simulink model "Target_Control_System"  (R2021b)
settings: Solver=FixedStepDiscrete  StartTime=0.0  StopTime=5  RelTol=1e-3
PreLoadFcn:
  | RTWConfigurationCB('preloadfcn', bdroot);
PostLoadFcn:
  | load('configuration/data_struct.mat');
  | load('configuration/fluxMaps_propMotor.mat');
  | load('configuration/parameterInit_PROP.mat');
  | load('configuration/parameterInit_PUMP.mat');
  | load('configuration/parameterInit_PITCH.mat');
  | load('configuration/parameterInit_TILT.mat');
  | %load('configuration/base_workspace_signal_definition.mat');
  | %load('resolvedatastores_to_baseworkspace_for_faster_simulation.mat');
model workspace (MAT data in the model file):
  SIMULATION_OPTIONS : Simulink.Parameter (value not decoded)
  TARGET_CODE_GEN : Simulink.Parameter (value not decoded)
  TCS_SAMPLE_FREQ_HZ : Simulink.Parameter (value not decoded)
symbols that are objects in the model workspace (value not decoded): TARGET_CODE_GEN, TCS_SAMPLE_FREQ_HZ
undefined symbols (not defined in the file): A_DQ_REF_LPF_INIT__PITCH, A_DQ_REF_LPF_INIT__PROP, A_DQ_REF_LPF_INIT__PUMP, A_DQ_REF_LPF_INIT__TILT, A_OBSERVER_CONFIDENCE_INIT__PITCH, A_OBSERVER_CONFIDENCE_INIT__PROP, A_OBSERVER_CONFIDENCE_INIT__PUMP, A_OBSERVER_CONFIDENCE_INIT__TILT, ACTUATOR_MAX_ANGLE_TRIP__PITCH, ACTUATOR_MIN_ANGLE_TRIP__PITCH, ACTUATOR_POS_SENSOR_INV_DIRECTION__PITCH, ACTUATOR_POS_SENSOR_INV_DIRECTION__TILT, ACTUATOR_POS_SENSOR_OFFSET__PITCH, ACTUATOR_POS_SENSOR_OFFSET__TILT, ADC_scaler1_baseaddr_TILT, ADC_SCALER_FLOAT_TO_FIXPOINT_EXPANSION, ANGLE_ELEC_FROM_SENSOR_OFFSET_INIT__PITCH, ANGLE_ELEC_FROM_SENSOR_OFFSET_INIT__PROP, ANGLE_ELEC_FROM_SENSOR_OFFSET_INIT__PUMP, ANGLE_ELEC_FROM_SENSOR_OFFSET_INIT__TILT, AUTO_CLEAR_FAULTS_ENABLED__PITCH, AUTO_CLEAR_FAULTS_ENABLED__PROP, AUTO_CLEAR_FAULTS_ENABLED__PUMP, AUTO_CLEAR_FAULTS_ENABLED__TILT, AUTO_CLEAR_FAULTS_WAIT_TICKS__PITCH, AUTO_CLEAR_FAULTS_WAIT_TICKS__PROP, AUTO_CLEAR_FAULTS_WAIT_TICKS__PUMP, AUTO_CLEAR_FAULTS_WAIT_TICKS__TILT, AUTO_I_ZERO_IDLE_TICKS__PITCH, AUTO_I_ZERO_IDLE_TICKS__PROP, AUTO_I_ZERO_IDLE_TICKS__PUMP, AUTO_I_ZERO_IDLE_TICKS__TILT, AUTO_I_ZERO_OFFSET_IDC_THRESHOLD__PITCH, AUTO_I_ZERO_OFFSET_IDC_THRESHOLD__PROP, AUTO_I_ZERO_OFFSET_IDC_THRESHOLD__PUMP, AUTO_I_ZERO_OFFSET_IDC_THRESHOLD__TILT, AUTO_I_ZERO_OFFSET_IPH_THRESHOLD__PITCH, AUTO_I_ZERO_OFFSET_IPH_THRESHOLD__PROP, AUTO_I_ZERO_OFFSET_IPH_THRESHOLD__PUMP, AUTO_I_ZERO_OFFSET_IPH_THRESHOLD__TILT, AUTO_SENSORLESS_SWITCHOVER_DISABLE_OMEGA, AUTO_SENSORLESS_SWITCHOVER_ENABLE_OMEGA, AUTO_SENSORLESS_SWITCHOVER_MIN_CONFIDENCE, AUXILIARY_PROTECTION_UNIT_BASEADDR__TILT, blanking_max_error_omega_INIT_PITCH, blanking_max_error_omega_INIT_TILT, blanking_max_error_position_INIT_PITCH, blanking_max_error_position_INIT_TILT, BRUTE_START_I_Q_REF_RAMP_SPEED__PITCH, BRUTE_START_I_Q_REF_RAMP_SPEED__PROP, BRUTE_START_I_Q_REF_RAMP_SPEED__PUMP, BRUTE_START_I_Q_REF_RAMP_SPEED__TILT, CONTROL_LOOP_DT_INIT__PITCH, CONTROL_LOOP_DT_INIT__PROP, CONTROL_LOOP_DT_INIT__PUMP, CONTROL_LOOP_DT_INIT__TILT, CORRECTION_FILTER_SCALE__PITCH, CORRECTION_FILTER_SCALE__PROP, CORRECTION_FILTER_SCALE__PUMP, CORRECTION_FILTER_SCALE__TILT ... (+458)
libraries: simulink x178, Reusables_Lib x24
(part 43 of 47)

== stateflow chart Target_Control_System/MainLoop/pumpMotor_mainLoop/motorStateMachineLogic(&oPump)/Idle-Loop State Machine Pump ==
  state InitialState
  state State_90
    //startup delay
    state Wait_Ticks_
    state Startup_Delay_
      entry:
      oPump.oMot_.oState_.uiDriveState_ = 95;
      oPump.oMot_.oOut_.uiLastFaultState_ = 0;
    (default) -> State_90.Wait_Ticks_
    State_90.Wait_Ticks_ -> Startup_Delay_ : [after(35, tick)]
  state State_246
    // Second phase of voltage nulling
    state Wait_uiDelayTicks_
    state Next
      entry:
      oPump.oMot_.oState_.uiDriveState_ = 100;
      oPump.oMot_.oOut_.uiEnableGateDrive_ = 0x0;
      oPump.oMot_.oIn_.uiVoltageOffsetNullingActive_ = 0;
    (default) -> State_246.Wait_uiDelayTicks_
    State_246.Wait_uiDelayTicks_ -> State_246.Next : [after(25, tick)]
  state State_95
    // Current offset nulling
    state Wait_Ticks_
    state Current_offset_nulling
      entry:
      oPump.oMot_.oState_.uiCurrentOffsetNullingPerformed_++;
      oPump.oMot_.oIn_.uiCurrentOffsetNullingActive_ = 0;
      oPump.oMot_.oIn_.uiVoltageOffsetNullingActive_ = 0;
      oPump.oMot_.oState_.uiDriveState_ = 99;
      //SZ: still need to re-write the FPGA protection to enable the sum of current detection for fault 1034
    (default) -> State_95.Wait_Ticks_
    State_95.Wait_Ticks_ -> Current_offset_nulling : [after(6, tick)]
  state State_245
    // Initial phase of voltage nulling
    state Wait_uiDelayTicks_
    state Next
      entry:
      oPump.oMot_.oState_.uiDriveState_ = 246;
    (default) -> State_245.Wait_uiDelayTicks_
    State_245.Wait_uiDelayTicks_ -> State_245.Next : [after(25, tick)]
  state State_99
    // Minimum command set not met. Also the return state after clearing trips etc.
    state Substate
    state Idle_state
      entry:
      oPump.oMot_.oState_.uiDriveState_ = 100;
    state Cleanup
      // We somehow left the forced angle start sequence without cleaning up.
      // Clean up now.
      entry:
      oPump.oMot_.oState_.oRampDataOmegaERef_.oParam_.fUpslope_ = oPump.oMot_.oState_.fForcedAngleStartOrigOmegaRamp_;
      oPump.oMot_.oState_.oRampDataOmegaERef_.fSetpoint_ = fabs(oPump.oMot_.oState_.fForcedAngleStartOrigOmega_);
      oPump.oMot_.oState_.uiSpeedControllerActive_ = oPump.oMot_.oState_.uiForcedAngleStartOrigSpeedControllerActive_;
      oPump.oMot_.oState_.oRampDataIqRef_.oParam_.fUpslope_ = oPump.oMot_.oState_.fForcedAngleStartOrigIRamp_;
      oPump.oMot_.oState_.oRampDataIqRef_.oParam_.fDownslope_ = oPump.oMot_.oState_.oRampDataIqRef_.oParam_.fUpslope_;
      oPump.oMot_.oOut_.uiForcedAngle_ = 0;
      oPump.oMot_.oState_.uiForcedAngleStartParametersSet_ = 0;
    (default) -> State_99.Substate
    State_99.Substate -> (junction 251)
    (junction 251) -> Idle_state [order 2] : [!oPump.oMot_.oState_.uiMinimumCommandSetFlags_]
    (junction 251) -> State_99.Cleanup [order 1] : [oPump.oMot_.oState_.uiForcedAngleStartParametersSet_]
    State_99.Cleanup -> Idle_state : [!oPump.oMot_.oState_.uiMinimumCommandSetFlags_]
  state State_104
    // Idle, motor spinning (windmilling, coasting down),
    // autostart enabled, and a nonzero current applied
    // Removed autostart functionality
    entry:
    oPump.oMot_.oState_.uiDriveState_ = 102;
  state State_224
    state Transition_220
      // Direction or confidence check failed, restart full sequence
      entry:
      oPump.oMot_.oState_.uiDriveState_ = 220;
    state FlyingStart
      entry:
      oPump.oMot_.oOut_.uiPwmDutyTicksFromMainA_ = uint32((oPump.oMot_.oParam_.fPwmPeriodTicksMainloopFloat_)/2);
      oPump.oMot_.oOut_.uiPwmDutyTicksFromMainB_ = uint32((oPump.oMot_.oParam_.fPwmPeriodTicksMainloopFloat_)/2);
      oPump.oMot_.oOut_.uiPwmDutyTicksFromMainC_ = uint32((oPump.oMot_.oParam_.fPwmPeriodTicksMainloopFloat_)/2);
      oPump.oMot_.oState_.oRampDataOmegaERef_.fRampOut_ = oPump.oMot_.oIn_.fOmegaEObserverLpf2_;
      oPump.oMot_.oState_.oRampDataIqRef_.fRampOut_ = 0.0;
      oPump.oIsr_.oParam_.oPiDataIq_.fState_ = 0.0F;
      oPump.oIsr_.oParam_.oPiDataId_.fState_ = 0.0F;
      oPump.oMot_.oParam_.oPiDataRpm_.fState_ = 0.0F;
      oPump.oMot_.oParam_.oPid2DataRpmCtrl_.fState_ = 0.0F;
      oPump.oMot_.oState_.uiDriveState_ = 200;
      // release gate signals
      oPump.oMot_.oOut_.uiEnableGateDrive_ = 0x7;
      // Release control in main interrupt
      oPump.oMot_.oOut_.uiCurrentControllerActive_ = 1;
    state uiAutomaticFanControlMode_
      entry:
      oPump.oMot_.oState_.uiDriveState_ = 205;
    (default) -> (junction 274)
    (junction 274) -> (junction 275) [order 2]
    (junction 274) -> (junction 276) [order 1] : [oPump.oMot_.oState_.fObserverConfidence_ > oPump.oMot_.oParam_.fSlaveStartMinConfidence_ && ....
        | !(oPump.oMot_.oOut_.fOmegaEObserverXlpf2_ * oPump.oMot_.oState_.fForcedAngleStartDirection_ < 0.0F)]
        | // The faster we go, the further we jump in the sequence
        | // [SZ]: need to investigate implementing the __signbitf() function in Stateflow]
    (junction 275) -> State_224.Transition_220
    (junction 276) -> FlyingStart : //Confidence wise we're good to go, but is the speed high enough?
        | [fabs(oPump.oMot_.oOut_.fOmegaEObserverXlpf2_) > ....
        |  (oPump.oMot_.oParam_.fSlaveStartMinOmegaE_)]
    FlyingStart -> State_224.uiAutomaticFanControlMode_ : [oPump.oMot_.oParam_.uiAutomaticFanControlMode_ == 1]
  state State_103
    // Idle, motor not spinning, autostart enabled, and a nonzero current applied
    // Removed autostart functionality
    entry:
    oPump.oMot_.oState_.uiDriveState_ = 101;
  state State_100
    //Idle, determine if the motor is externally driven (e.g. windmilling or spindown) or standing still
    state Initialization
      entry:
      oPump.oMot_.oState_.oRampDataOmegaERef_.fRampOut_ = 0.0;
      oPump.oMot_.oState_.oRampDataIqRef_.fRampOut_ = 0.0;
    state Entering_State_101
      entry:
      oPump.oMot_.oState_.uiDriveState_ = 101;
    state Cleanup
      // We somehow left the forced angle start sequence without cleaning up.
      // Clean up now.
      entry:
      oPump.oMot_.oState_.uiDriveState_  = 99;
    state Entering_State_102
      entry:
      oPump.oMot_.oState_.uiDriveState_ = 102;
    state pwm50PercentDuty
      //Pre-set 50% duty
      entry:
      oPump.oMot_.oOut_.uiPwmRequestFromMain_ = 1;
      oPump.oMot_.oOut_.uiPwmDutyTicksFromMainA_ = cast(((oPump.oMot_.oParam_.fPwmPeriodTicksMainloopFloat_) / 2), uint32);
      oPump.oMot_.oOut_.uiPwmDutyTicksFromMainB_ = cast(((oPump.oMot_.oParam_.fPwmPeriodTicksMainloopFloat_) / 2), uint32);
      oPump.oMot_.oOut_.uiPwmDutyTicksFromMainC_ = cast(((oPump.oMot_.oParam_.fPwmPeriodTicksMainloopFloat_) / 2), uint32);
    (default) -> State_100.Initialization
    State_100.Initialization -> (junction 189)
    (junction 189) -> (junction 186) [order 2]
    (junction 186) -> Entering_State_101 [order 1] : [(fabs(oPump.oMot_.oOut_.fOmegaEObserverXlpf2_) < oPump.oMot_.oParam_.fFlyingStartOmegaELimit_) ....
        |  || (oPump.oMot_.oState_.fObserverConfidence_ < 0.7F)]
    (junction 189) -> State_100.Cleanup [order 1] : [oPump.oMot_.oState_.uiMinimumCommandSetFlags_]
    (junction 186) -> Entering_State_102 [order 2]
    Entering_State_101 -> pwm50PercentDuty
    Entering_State_102 -> pwm50PercentDuty
  state State_102
    // Idle, motor spinning by external means (windmilling, downhill, large inertia, ....)
    state Stay_at_102
      entry:
      oPump.oMot_.oState_.uiDriveState_ = 102;
    state Transition_to_101
      entry:
      oPump.oMot_.oState_.uiDriveState_ = 101;
    (default) -> (junction 192)
    (junction 192) -> Stay_at_102 [order 2]
    (junction 192) -> Transition_to_101 [order 1] : [fabs(oPump.oMot_.oOut_.fOmegaEObserverXlpf2_) < oPump.oMot_.oParam_.fFlyingStartOmegaELimit_ ....
        | || oPump.oMot_.oState_.fObserverConfidence_ < 0.65F]
  state State_222
    state Transition_224
      entry:
      oPump.oMot_.oState_.uiDriveState_ = 224;
    state Transition_223
      entry:
      oPump.oMot_.oState_.uiDriveState_ = 223;
    state Transition_220
      // Direction or confidence check failed, restart full sequence
      entry:
      oPump.oMot_.oState_.uiDriveState_ = 220;
    (default) -> (junction 301)
    (junction 301) -> (junction 302) [order 2]
    (junction 301) -> (junction 304) [order 1] : [oPump.oMot_.oState_.fObserverConfidence_ > oPump.oMot_.oParam_.fSlaveStartMinConfidence_ && ....
        | !(oPump.oMot_.oOut_.fOmegaEObserverXlpf2_ * oPump.oMot_.oState_.fForcedAngleStartDirection_ < 0.0F)]
        | // The faster we go, the further we jump in the sequence
        | // [SZ]: need to investigate implementing the __signbitf() function in Stateflow]
    (junction 302) -> State_222.Transition_220
    (junction 304) -> (junction 303) [order 1]
    (junction 303) -> State_222.Transition_224 : [fabs(oPump.oMot_.oOut_.fOmegaEObserverXlpf2_) >....
        |  (oPump.oMot_.oParam_.fSlaveStartMinOmegaE_)]
    (junction 304) -> State_222.Transition_223 [order 2]
  state State_223
    state Transition_220
      // Direction or confidence check failed, restart full sequence
      entry:
      oPump.oMot_.oState_.uiDriveState_ = 220;
    state Transition_224
      entry:
      oPump.oMot_.oState_.uiDriveState_ = 224;
    (default) -> (junction 263)
    (junction 263) -> (junction 264) [order 2]
    (junction 263) -> (junction 265) [order 1] : [oPump.oMot_.oState_.fObserverConfidence_ > oPump.oMot_.oParam_.fSlaveStartMinConfidence_ && ....
        | !(oPump.oMot_.oOut_.fOmegaEObserverXlpf2_ * oPump.oMot_.oState_.fForcedAngleStartDirection_ < 0.0F)]
        | // The faster we go, the further we jump in the sequence
        | // [SZ]: need to investigate implementing the __signbitf() function in Stateflow]
    (junction 264) -> State_223.Transition_220
    (junction 265) -> State_223.Transition_224 : [fabs(oPump.oMot_.oOut_.fOmegaEObserverXlpf2_) >....
        |  (oPump.oMot_.oParam_.fSlaveStartMinOmegaE_)]
  state State_101
    // Idle, motor not spinning
    state Initialization
      entry:
      oPump.oMot_.oState_.oRampDataOmegaERef_.fRampOut_ = 0.0;
      oPump.oMot_.oState_.oRampDataIqRef_.fRampOut_ = 0.0;
    state Transition_to_102
      entry:
      oPump.oMot_.oState_.uiDriveState_ = 102;
    (default) -> State_101.Initialization
    State_101.Initialization -> (junction 227)
    (junction 227) -> Transition_to_102 [order 1] : [(fabs(oPump.oMot_.oOut_.fOmegaEObserverXlpf2_) > oPump.oMot_.oParam_.fFlyingStartOmegaELimit_) ....
        | && (oPump.oMot_.oState_.fObserverConfidence_ > 0.65F)]
  state State_220
    // Flying start, first of multiple stages.
    // There has to be an uninterrupted chain of OKs. Too low confidence at any step,
    // and fall back to this initial state.
    state Substate
    state Transition_224
      entry:
      oPump.oMot_.oState_.uiDriveState_ = 224;
    state Transition_223
      entry:
      oPump.oMot_.oState_.uiDriveState_ = 223;
    state Transition_222
      entry:
      oPump.oMot_.oState_.uiDriveState_ = 222;
    state Transition_221
      /* Don't check for the speed for the slowest
      //advancement path, that will happen in state 224 */
      entry:
      oPump.oMot_.oState_.uiDriveState_ = 221;
    (default) -> State_220.Substate
    State_220.Substate -> (junction 346)
    (junction 346) -> (junction 348) : [oPump.oMot_.oState_.fObserverConfidence_ > oPump.oMot_.oParam_.fSlaveStartMinConfidence_ && ....
        | !(oPump.oMot_.oOut_.fOmegaEObserverXlpf2_ * oPump.oMot_.oState_.fForcedAngleStartDirection_ < 0.0F)]
        | // The faster we go, the further we jump in the sequence
        | // [SZ]: need to investigate implementing the __signbitf() function in Stateflow]
    (junction 348) -> (junction 347) [order 1]
    (junction 348) -> (junction 349) [order 3]
    (junction 349) -> (junction 350) [order 2]
    (junction 347) -> State_220.Transition_224 : [fabs(oPump.oMot_.oOut_.fOmegaEObserverXlpf2_) >....
        |  (oPump.oMot_.oParam_.fSlaveStartMinOmegaE_)]
    (junction 348) -> State_220.Transition_223 [order 2] : [fabs(4.0F * oPump.oMot_.oOut_.fOmegaEObserverXlpf2_) >....
        |  (3.0F * oPump.oMot_.oParam_.fSlaveStartMinOmegaE_)]
    (junction 349) -> State_220.Transition_222 [order 1] : [fabs(2.0F * oPump.oMot_.oOut_.fOmegaEObserverXlpf2_) >....
        |  (oPump.oMot_.oParam_.fSlaveStartMinOmegaE_)]
    (junction 350) -> Transition_221
  state State_221
    state Transition_224
      entry:
      oPump.oMot_.oState_.uiDriveState_ = 224;
    state Transition_223
      entry:
      oPump.oMot_.oState_.uiDriveState_ = 223;
    state Transition_222
      entry:
      oPump.oMot_.oState_.uiDriveState_ = 222;
    state Transition_220
      // Direction or confidence check failed, restart full sequence
      entry:
      oPump.oMot_.oState_.uiDriveState_ = 220;
    (default) -> (junction 298)
    (junction 298) -> (junction 328) [order 2]
    (junction 298) -> (junction 330) [order 1] : [oPump.oMot_.oState_.fObserverConfidence_ > oPump.oMot_.oParam_.fSlaveStartMinConfidence_ && ....
        | !(oPump.oMot_.oOut_.fOmegaEObserverXlpf2_ * oPump.oMot_.oState_.fForcedAngleStartDirection_ < 0.0F)]
        | // The faster we go, the further we jump in the sequence
        | // [SZ]: need to investigate implementing the __signbitf() function in Stateflow]
    (junction 328) -> State_221.Transition_220
    (junction 330) -> (junction 329) [order 1]
    (junction 330) -> (junction 331) [order 3]
    (junction 329) -> State_221.Transition_224 : [fabs(oPump.oMot_.oOut_.fOmegaEObserverXlpf2_) >....
        |  (oPump.oMot_.oParam_.fSlaveStartMinOmegaE_)]
    (junction 330) -> State_221.Transition_223 [order 2] : [fabs(4.0F * oPump.oMot_.oOut_.fOmegaEObserverXlpf2_) >....
        |  (3.0F * oPump.oMot_.oParam_.fSlaveStartMinOmegaE_)]
    (junction 331) -> State_221.Transition_222
  state State_212
    // Forced angle. Current and speed are ramping.
    // Once we reach a certain predefined speed, turn off forced angle
    // (idea: look at observer confidence instead, or additionally)
    state Wait_RPM
      exit:
      // To avoid a sudden step in angle, add an offset to the estimated angle to give the forced angle. It'll ramp to zero
      //oPump.oMot_.oState_.oRampDataFluxMstrAngFrcd2clsdSmoothn_.fRampOut_ = oPump.oIsr_.oState_.fFluxMasterAngle_ - oPump.oIsr_.oState_.fFluxMainAngleRaw2_;
    state Restore_values
      // Restore values: (Mind the order of setting things, in case the interrupt starts halfway through)
      state Reset
        entry:
        oPump.oMot_.oOut_.uiForcedAngle_ = 0;
        oPump.oMot_.oState_.oRampDataOmegaERef_.oParam_.fUpslope_ = oPump.oMot_.oState_.fForcedAngleStartOrigOmegaRamp_;
        // The downslope wasn't touched in the first place, as forced angle start only relies on the upslope
        oPump.oMot_.oState_.uiDriveState_ = 213;
      (default) -> (junction 434)
      (junction 434) -> (junction 437) [order 1] : [oPump.oMot_.oState_.oRampDataFluxMstrAngFrcd2clsdSmoothn_.fRampOut_> PI_F]
          | {oPump.oMot_.oState_.oRampDataFluxMstrAngFrcd2clsdSmoothn_.fRampOut_ -= TWO_PI_F;}
      (junction 437) -> Reset [order 2]
      (junction 434) -> Reset [order 3]
      (junction 434) -> Reset [order 2] : [oPump.oMot_.oState_.oRampDataFluxMstrAngFrcd2clsdSmoothn_.fRampOut_ < -PI_F]
          | {oPump.oMot_.oState_.oRampDataFluxMstrAngFrcd2clsdSmoothn_.fRampOut_ += TWO_PI_F;}
      (junction 437) -> Reset [order 1] : [oPump.oMot_.oState_.oRampDataFluxMstrAngFrcd2clsdSmoothn_.fRampOut_ < -PI_F]
          | {oPump.oMot_.oState_.oRampDataFluxMstrAngFrcd2clsdSmoothn_.fRampOut_ += TWO_PI_F;}
    (default) -> Wait_RPM
    Wait_RPM -> Restore_values : [oPump.oMot_.oState_.oRampDataOmegaERef_.fRampOut_ > oPump.oMot_.oParam_.fForcedAngleOmegaEHandoff_ ]
  state State_213
    // Almost the end of forced angle
    state Wait_uiForcedStartPostTicks_
      exit:
      oPump.oMot_.oState_.oRampDataIqRef_.oParam_.fUpslope_ = oPump.oMot_.oState_.fForcedAngleStartOrigIRamp_;	// TODO whatabout downslope
      oPump.oMot_.oState_.oRampDataIqRef_.oParam_.fDownslope_ = oPump.oMot_.oState_.oRampDataIqRef_.oParam_.fUpslope_;
      oPump.oMot_.oState_.uiForcedAngleStartParametersSet_ = 0;
      oPump.oMot_.oState_.uiDriveState_ = 200;
    state uiAutomaticFanControlMode_
      entry:
      oPump.oMot_.oState_.uiDriveState_ = 205;
    (default) -> Wait_uiForcedStartPostTicks_
    Wait_uiForcedStartPostTicks_ -> (junction 409) : [after(oPump.oMot_.oParam_.uiForcedStartPostTicks_, tick)]
    (junction 409) -> (junction 406) [order 2]
    (junction 409) -> State_213.uiAutomaticFanControlMode_ [order 1] : [oPump.oMot_.oParam_.uiAutomaticFanControlMode_ == 1]
    State_213.uiAutomaticFanControlMode_ -> (junction 406)
  state State_211
    // Forced angle start, ramping the current while holding speed at zero.
    // After some time, we release the speed
    state Wait_uiForcedAngleSpeedDelayTicks_
    state Speed_loop_active
      entry:
      oPump.oMot_.oState_.oRampDataOmegaERef_.fSetpoint_ = oPump.oMot_.oState_.fForcedAngleStartOrigOmega_;
    state Speed_loop_inactive
      // Torque control. We don't actually know if the current is enough to reach the handoff point
      // So, we set the speedref to a bit above the handoff point. Past the handoff, this value becomes irrelevant.
      entry:
      oPump.oMot_.oState_.oRampDataOmegaERef_.fSetpoint_ = oPump.oMot_.oParam_.fForcedAngleOmegaEHandoff_ * 1.1F;
    state Bidirection
      // allow for clock and counterclockwise dir depending on current setpoint
      entry:
      oPump.oMot_.oState_.oRampDataOmegaERef_.fSetpoint_ = abs(oPump.oMot_.oState_.oRampDataOmegaERef_.fSetpoint_) * oPump.oMot_.oState_.fForcedAngleStartDirection_;
      oPump.oMot_.oState_.uiDriveState_ = 212;
    (default) -> Wait_uiForcedAngleSpeedDelayTicks_
    Wait_uiForcedAngleSpeedDelayTicks_ -> (junction 375) : [after(oPump.oMot_.oParam_.uiForcedAngleSpeedDelayTicks_, tick)]
    (junction 375) -> Speed_loop_active [order 1] : [oPump.oMot_.oState_.uiSpeedControllerActive_ == 1]
    (junction 375) -> Speed_loop_inactive [order 2]
    Speed_loop_active -> Bidirection
    Speed_loop_inactive -> Bidirection
  (default) -> InitialState
  InitialState -> State_90 [order 1] : [oPump.oMot_.oState_.uiDriveState_ == 90]
  State_90 -> InitialState : [!(oPump.oMot_.oState_.uiDriveState_ == 90)]
  InitialState -> State_246 [order 12] : [oPump.oMot_.oState_.uiDriveState_ == 246]
  State_246 -> InitialState : [!(oPump.oMot_.oState_.uiDriveState_ == 246)]
  InitialState -> State_95 [order 2] : [oPump.oMot_.oState_.uiDriveState_ == 95]
  Current_offset_nulling -> InitialState : [!(oPump.oMot_.oState_.uiDriveState_ == 95)]
  InitialState -> State_245 [order 11] : [oPump.oMot_.oState_.uiDriveState_ == 245]
  State_245 -> InitialState : [!(oPump.oMot_.oState_.uiDriveState_ == 245)]
  InitialState -> State_99 [order 3] : [oPump.oMot_.oState_.uiDriveState_ == 99]
  State_99 -> InitialState : [!(oPump.oMot_.oState_.uiDriveState_ == 99)]
  InitialState -> State_104 [order 8] : [oPump.oMot_.oState_.uiDriveState_ == 104]
  State_104 -> InitialState
  InitialState -> State_103 [order 7] : [oPump.oMot_.oState_.uiDriveState_ == 103]
  State_103 -> InitialState
  InitialState -> State_102 [order 6] : [oPump.oMot_.oState_.uiDriveState_ == 102]
  Stay_at_102 -> InitialState
  State_100.Cleanup -> InitialState
  Transition_to_101 -> InitialState
  pwm50PercentDuty -> InitialState
  InitialState -> State_100 [order 4] : [oPump.oMot_.oState_.uiDriveState_ == 100]
  InitialState -> State_101 [order 5] : [oPump.oMot_.oState_.uiDriveState_ == 101]
  State_224 -> (junction 293) : [!(oPump.oMot_.oState_.uiDriveState_ == 224)]
  (junction 293) -> State_224 [order 4] : [oPump.oMot_.oState_.uiDriveState_ == 224]
  State_223 -> (junction 293) : [!(oPump.oMot_.oState_.uiDriveState_ == 223)]
  (junction 293) -> State_223 [order 3] : [oPump.oMot_.oState_.uiDriveState_ == 223]
  State_222 -> (junction 293) : [!(oPump.oMot_.oState_.uiDriveState_ == 222)]
  (junction 322) -> State_222 [order 2] : [oPump.oMot_.oState_.uiDriveState_ == 222]
  (junction 227) -> InitialState [order 2] : // We're staying at rest.
  Transition_to_102 -> InitialState
  InitialState -> (junction 293) [order 10] : [(oPump.oMot_.oState_.uiDriveState_ >= 220) && (oPump.oMot_.oState_.uiDriveState_ <= 224)]
  (junction 293) -> InitialState [order 5]
  (junction 293) -> (junction 322) [order 2]
  State_221 -> (junction 293) : [!(oPump.oMot_.oState_.uiDriveState_ == 221)]
  State_220 -> (junction 293) : [!(oPump.oMot_.oState_.uiDriveState_ == 220)]
  (junction 293) -> State_220 [order 1] : [oPump.oMot_.oState_.uiDriveState_ == 220]
  (junction 322) -> State_221 [order 1] : [oPump.oMot_.oState_.uiDriveState_ == 221]
  InitialState -> (junction 380) [order 9] : [oPump.oMot_.oState_.uiDriveState_ == 211]
  (junction 380) -> InitialState [order 4]
  (junction 406) -> (junction 380) : {oPump.oMot_.oState_.oRampDataIqRef_.oParam_.fUpslope_ = oPump.oMot_.oState_.fForcedAngleStartOrigIRamp_;
      |  oPump.oMot_.oState_.oRampDataIqRef_.oParam_.fDownslope_ = oPump.oMot_.oState_.oRampDataIqRef_.oParam_.fUpslope_;
      |  oPump.oMot_.oState_.uiForcedAngleStartParametersSet_ = 0;}
  State_212 -> (junction 380) : [!(oPump.oMot_.oState_.uiDriveState_ == 212)]
      | {oPump.oMot_.oState_.oRampDataOmegaERef_.oParam_.fUpslope_ = oPump.oMot_.oState_.fForcedAngleStartOrigOmegaRamp_;
      | oPump.oMot_.oState_.oRampDataOmegaERef_.fSetpoint_ = fabs(oPump.oMot_.oState_.fForcedAngleStartOrigOmega_);
      | oPump.oMot_.oState_.oRampDataOmegaERef_.fRampOut_ = oPump.oMot_.oOut_.fOmegaEObserverXlpf2_;  // For the speed controller, if used
      | oPump.oMot_.oState_.uiSpeedControllerActive_ = oPump.oMot_.oState_.uiForcedAngleStartOrigSpeedControllerActive_;
      | oPump.oMot_.oOut_.uiForcedAngle_ = 0;}
  (junction 380) -> State_212 [order 2] : [oPump.oMot_.oState_.uiDriveState_ == 212]
  (junction 380) -> State_213 [order 3] : [oPump.oMot_.oState_.uiDriveState_ == 213]
  State_211 -> (junction 380) : [!(oPump.oMot_.oState_.uiDriveState_ == 211)]
  (junction 380) -> State_211 [order 1] : [oPump.oMot_.oState_.uiDriveState_ == 211]
  data: oPump data_store_memory; PI_F constant single =3.14159265359; TWO_PI_F constant single =6.28318530718

== stateflow chart Target_Control_System/MainLoop/pumpMotor_mainLoop/Decimation gate A for 200 Hz Pump/Current offset nulling/initiateOffsetNulling(&oPump)/Chart ==
  state Start
  state initiateOffsetNulling
    //We can only do this if idle
    entry:
    oPump.oIsr_.oState_.fOffsetIntegratorIa_ = 0.0;
    oPump.oIsr_.oState_.fOffsetIntegratorIb_ = 0.0;
    oPump.oIsr_.oState_.fOffsetIntegratorIc_ = 0.0;
    oPump.oIsr_.oState_.fOffsetIntegratorIdc_ = 0.0;
    oPump.oMot_.oState_.uiDriveState_ = 95;
  (default) -> Start
  initiateOffsetNulling -> Start : [oPump.oMot_.oState_.uiCurrentOffsetNullingPerformed_ == 1]
  Start -> initiateOffsetNulling : [oPump.oMot_.oState_.uiDriveState_ >= 99 && ...
      | oPump.oMot_.oState_.uiDriveState_ < 102]
  data: oPump data_store_memory

== stateflow chart Target_Control_System/MainLoop/pitchMotor_mainLoop/Decimation gate for 10 Hz Pitch/Idle-Loop State Machine Pitch ==
  state InitialState
  state State_90
    //startup delay
    state Wait_Ticks_
    state Startup_Delay_
      entry:
      oPitch.oMot_.oState_.uiDriveState_ = 95;
      oPitch.oMot_.oOut_.uiLastFaultState_ = 0;
    (default) -> State_90.Wait_Ticks_
    State_90.Wait_Ticks_ -> Startup_Delay_ : [after(35, tick)]
  state State_246
    // Second phase of voltage nulling
    state Wait_uiDelayTicks_
    state Next
      entry:
      oPitch.oMot_.oState_.uiDriveState_ = 100;
      oPitch.oMot_.oOut_.uiEnableGateDrive_ = 0x0;
      oPitch.oMot_.oIn_.uiVoltageOffsetNullingActive_ = 0;
    (default) -> State_246.Wait_uiDelayTicks_
    State_246.Wait_uiDelayTicks_ -> State_246.Next : [after(25, tick)]
  state State_95
    // Current offset nulling
    state Wait_Ticks_
    state Current_offset_nulling
      entry:
      oPitch.oMot_.oState_.uiCurrentOffsetNullingPerformed_++;
      oPitch.oMot_.oIn_.uiCurrentOffsetNullingActive_ = 0;
      oPitch.oMot_.oIn_.uiVoltageOffsetNullingActive_ = 0;
      oPitch.oMot_.oState_.uiDriveState_ = 99;
      //SZ: still need to re-write the FPGA protection to enable the sum of current detection for fault 1034
    (default) -> State_95.Wait_Ticks_
    State_95.Wait_Ticks_ -> Current_offset_nulling : [after(6, tick)]
  state State_245
    // Initial phase of voltage nulling
    state Wait_uiDelayTicks_
    state Next
      entry:
      oPitch.oMot_.oState_.uiDriveState_ = 246;
    (default) -> State_245.Wait_uiDelayTicks_
    State_245.Wait_uiDelayTicks_ -> State_245.Next : [after(25, tick)]
  state State_99
    // Minimum command set not met. Also the return state after clearing trips etc.
    state Substate
    state Idle_state
      entry:
      oPitch.oMot_.oState_.uiDriveState_ = 100;
    state Cleanup
      // We somehow left the forced angle start sequence without cleaning up.
      // Clean up now.
      entry:
      oPitch.oMot_.oState_.oRampDataOmegaERef_.oParam_.fUpslope_ = oPitch.oMot_.oState_.fForcedAngleStartOrigOmegaRamp_;
      oPitch.oMot_.oState_.oRampDataOmegaERef_.fSetpoint_ = fabs(oPitch.oMot_.oState_.fForcedAngleStartOrigOmega_);
      oPitch.oMot_.oState_.uiSpeedControllerActive_ = oPitch.oMot_.oState_.uiForcedAngleStartOrigSpeedControllerActive_;
      oPitch.oMot_.oState_.oRampDataIqRef_.oParam_.fUpslope_ = oPitch.oMot_.oState_.fForcedAngleStartOrigIRamp_;
      oPitch.oMot_.oState_.oRampDataIqRef_.oParam_.fDownslope_ = oPitch.oMot_.oState_.oRampDataIqRef_.oParam_.fUpslope_;
      oPitch.oMot_.oOut_.uiForcedAngle_ = 0;
      oPitch.oMot_.oState_.uiForcedAngleStartParametersSet_ = 0;
    (default) -> Substate
    Substate -> (junction 251)
    (junction 251) -> Idle_state [order 2] : [!oPitch.oMot_.oState_.uiMinimumCommandSetFlags_]
    (junction 251) -> State_99.Cleanup [order 1] : [oPitch.oMot_.oState_.uiForcedAngleStartParametersSet_]
    State_99.Cleanup -> Idle_state : [!oPitch.oMot_.oState_.uiMinimumCommandSetFlags_]
  state State_104
    // Idle, motor spinning (windmilling, coasting down),
    // autostart enabled, and a nonzero current applied
    // Removed autostart functionality
    entry:
    oPitch.oMot_.oState_.uiDriveState_ = 102;
  state State_103
    // Idle, motor not spinning, autostart enabled, and a nonzero current applied
    // Removed autostart functionality
    entry:
    oPitch.oMot_.oState_.uiDriveState_ = 101;
  state State_100
    //Idle, determine if the motor is externally driven (e.g. windmilling or spindown) or standing still
    state Initialization
      entry:
      oPitch.oMot_.oState_.oRampDataOmegaERef_.fRampOut_ = 0.0;
      oPitch.oMot_.oState_.oRampDataIqRef_.fRampOut_ = 0.0;
    state Entering_State_101
      entry:
      oPitch.oMot_.oState_.uiDriveState_ = 101;
    state Cleanup
      // We somehow left the forced angle start sequence without cleaning up.
      // Clean up now.
      entry:
      oPitch.oMot_.oState_.uiDriveState_  = 99;
    state Entering_State_102
      entry:
      oPitch.oMot_.oState_.uiDriveState_ = 102;
    state pwm50PercentDuty
      //Pre-set 50% duty
      entry:
      oPitch.oMot_.oOut_.uiPwmRequestFromMain_ = 1;
      oPitch.oMot_.oOut_.uiPwmDutyTicksFromMainA_ = cast(((oPitch.oMot_.oParam_.fPwmPeriodTicksMainloopFloat_) / 2), uint32);
      oPitch.oMot_.oOut_.uiPwmDutyTicksFromMainB_ = cast(((oPitch.oMot_.oParam_.fPwmPeriodTicksMainloopFloat_) / 2), uint32);
      oPitch.oMot_.oOut_.uiPwmDutyTicksFromMainC_ = cast(((oPitch.oMot_.oParam_.fPwmPeriodTicksMainloopFloat_) / 2), uint32);
    (default) -> State_100.Initialization
    State_100.Initialization -> (junction 189)
    (junction 189) -> (junction 186) [order 2]
    (junction 186) -> Entering_State_101 [order 1] : [(fabs(oPitch.oMot_.oOut_.fOmegaEObserverXlpf2_) < oPitch.oMot_.oParam_.fFlyingStartOmegaELimit_) ....
        |  || (oPitch.oMot_.oState_.fObserverConfidence_ < 0.7F)]
    (junction 189) -> State_100.Cleanup [order 1] : [oPitch.oMot_.oState_.uiMinimumCommandSetFlags_]
    (junction 186) -> Entering_State_102 [order 2]
    Entering_State_101 -> pwm50PercentDuty
    Entering_State_102 -> pwm50PercentDuty
  state State_102
    // Idle, motor spinning by external means (windmilling, downhill, large inertia, ....)
    state Stay_at_102
      entry:
      oPitch.oMot_.oState_.uiDriveState_ = 102;
    state Transition_to_101
      entry:
      oPitch.oMot_.oState_.uiDriveState_ = 101;
    (default) -> (junction 192)
    (junction 192) -> Stay_at_102 [order 2]
    (junction 192) -> Transition_to_101 [order 1] : [fabs(oPitch.oMot_.oOut_.fOmegaEObserverXlpf2_) < oPitch.oMot_.oParam_.fFlyingStartOmegaELimit_ ....
        | || oPitch.oMot_.oState_.fObserverConfidence_ < 0.65F]
  state State_101
    // Idle, motor not spinning
    state Initialization
      entry:
      oPitch.oMot_.oState_.oRampDataOmegaERef_.fRampOut_ = 0.0;
      oPitch.oMot_.oState_.oRampDataIqRef_.fRampOut_ = 0.0;
    state Transition_to_102
      entry:
      oPitch.oMot_.oState_.uiDriveState_ = 102;
    (default) -> State_101.Initialization
    State_101.Initialization -> (junction 227)
    (junction 227) -> Transition_to_102 [order 1] : [(fabs(oPitch.oMot_.oOut_.fOmegaEObserverXlpf2_) > oPitch.oMot_.oParam_.fFlyingStartOmegaELimit_) ....
        | && (oPitch.oMot_.oState_.fObserverConfidence_ > 0.65F)]
  (default) -> InitialState
  InitialState -> State_90 [order 1] : [oPitch.oMot_.oState_.uiDriveState_ == 90]
  State_90 -> InitialState : [!(oPitch.oMot_.oState_.uiDriveState_ == 90)]
  InitialState -> State_246 [order 10] : [oPitch.oMot_.oState_.uiDriveState_ == 246]
  State_246 -> InitialState : [!(oPitch.oMot_.oState_.uiDriveState_ == 246)]
  InitialState -> State_95 [order 2] : [oPitch.oMot_.oState_.uiDriveState_ == 95]
  Current_offset_nulling -> InitialState : [!(oPitch.oMot_.oState_.uiDriveState_ == 95)]
  InitialState -> State_245 [order 9] : [oPitch.oMot_.oState_.uiDriveState_ == 245]
  State_245 -> InitialState : [!(oPitch.oMot_.oState_.uiDriveState_ == 245)]
  InitialState -> State_99 [order 3] : [oPitch.oMot_.oState_.uiDriveState_ == 99]
  State_99 -> InitialState : [!(oPitch.oMot_.oState_.uiDriveState_ == 99)]
  InitialState -> State_104 [order 8] : [oPitch.oMot_.oState_.uiDriveState_ == 104]
  State_104 -> InitialState
  InitialState -> State_103 [order 7] : [oPitch.oMot_.oState_.uiDriveState_ == 103]
  State_103 -> InitialState
  InitialState -> State_102 [order 6] : [oPitch.oMot_.oState_.uiDriveState_ == 102]
  Stay_at_102 -> InitialState
  State_100.Cleanup -> InitialState
  Transition_to_101 -> InitialState
  pwm50PercentDuty -> InitialState
  InitialState -> State_100 [order 4] : [oPitch.oMot_.oState_.uiDriveState_ == 100]
  InitialState -> State_101 [order 5] : [oPitch.oMot_.oState_.uiDriveState_ == 101]
  (junction 227) -> InitialState [order 2] : // We're staying at rest.
  Transition_to_102 -> InitialState
  data: oPitch data_store_memory; PI_F constant single =3.14159265359; TWO_PI_F constant single =6.28318530718

== stateflow chart Target_Control_System/MainLoop/pitchMotor_mainLoop/Decimation gate for 10 Hz Pitch/Function-Call Subsystem/DC_overvoltage_pitch ==
  state Start
  state Drive_trip
    // Disable the drive and enter a trip state (error state)
    entry:
    oPitch.oMot_.oOut_.uiEnableGateDrive_ = 0;
    oPitch.oMot_.oOut_.uiCurrentControllerActive_ = 0;
    // NOTE: the actual turning off is done in the ctrl interrupt
    // formerly: Xil_Out32(uiGateDriverBaseaddr_, 0x0);
  state Store_previous_fault
    // If we were already in a fault state, store the previous fault:
    entry:
    oPitch.oMot_.oOut_.uiLastFaultState_ = oPitch.oMot_.oState_.uiDriveState_;
  state setTripState
    entry:
    oPitch.oMot_.oState_.uiDriveState_ = Udc_tripCode;
  (default) -> Start
  Start -> (junction 26) [order 2] : [(oPitch.oMot_.oOut_.fUdcLpf_ > oPitch.oMot_.oParam_.fUdcMaxTrip_) && ...
      | oPitch.oMot_.oState_.uiDriveState_ > 0]
      | {Udc_tripCode = 1004;}
  Start -> (junction 26) [order 1] : [oPitch.oMot_.oOut_.fUdcLpf_ < oPitch.oMot_.oParam_.fUdcMinTrip_ && ...
      | (oPitch.oMot_.oState_.uiDriveState_ > 199 && oPitch.oMot_.oState_.uiDriveState_ < 1000)]
      | {Udc_tripCode = 1003;}
  setTripState -> Start
  (junction 26) -> Drive_trip [order 1] : [oPitch.oMot_.oState_.uiDriveState_ >= 200]
  (junction 26) -> (junction 31) [order 2]
  Drive_trip -> (junction 31)
  (junction 31) -> Store_previous_fault [order 1] : [oPitch.oMot_.oState_.uiDriveState_ >= 1000]
  (junction 31) -> setTripState [order 2]
  Store_previous_fault -> setTripState
  data: Udc_tripCode local single; oPitch data_store_memory

== stateflow chart Target_Control_System/MainLoop/tiltMotor_mainLoop/mainTask_tilt/motorTaskMainFastStep(&oTilt)/enableDrive(&oTilt) ==
  state Disabled
    state Default
    state Disable_Drive
      entry:
      oTilt.oMot_.oState_.uiDriveState_ = 100;
      oTilt.oMot_.oOut_.uiEnableGateDrive_ = 0x0;
      oTilt.oMot_.oOut_.uiCurrentControllerActive_ = 0;
    state Simulation
      entry:
      oTilt.oMot_.oState_.uiDriveState_ = 101;
      oTilt.oMot_.oOut_.uiEnableGateDrive_ = 0x0;
    (default) -> (junction 283)
    (junction 283) -> Default [order 3]
    (junction 283) -> Disable_Drive [order 2] : [oTilt.oMot_.oState_.uiDriveState_ >= 200 && ....
        |  oTilt.oMot_.oState_.uiDriveState_ <= 299]
    (junction 283) -> Simulation [order 1] : [TARGET_CODE_GEN ==0]
  state Position_hold_mode
    // Mostly intended for the VP. In position hold mode, the inverter will inject 0 RPM current in the motor to passively hold a motor in place.
    // The position sensors are not needed for this.
    // When issuing the enable command, the drive enters state 226, which is just for flagging, the inverters do not actually turn on.
    // (Use a special command for that.)
    entry:
    oTilt.oMot_.oState_.uiDriveState_ = 226;
    oTilt.oIsr_.oParam_.oPiDataIq_.fState_ = 0;
    oTilt.oIsr_.oParam_.oPiDataId_.fState_ = 0;
    // Pre-set 50% duty
    oTilt.oMot_.oOut_.uiPwmRequestFromMain_ = 1;
    oTilt.oMot_.oOut_.uiPwmDutyTicksFromMainA_ = uint32((oTilt.oMot_.oParam_.fPwmPeriodTicksMainloopFloat_)/2);
    oTilt.oMot_.oOut_.uiPwmDutyTicksFromMainB_ = uint32((oTilt.oMot_.oParam_.fPwmPeriodTicksMainloopFloat_)/2);
    oTilt.oMot_.oOut_.uiPwmDutyTicksFromMainC_ = uint32((oTilt.oMot_.oParam_.fPwmPeriodTicksMainloopFloat_)/2);
  state DC_undervoltage_trip
    state Fault_A
      entry:
      oTilt.oMot_.oOut_.uiCurrentControllerActive_ = 0;
      oTilt.oMot_.oOut_.uiEnableGateDrive_ = 0;
    state Fault_B
      // If we were already in a fault state, store the previous fault:
      entry:
      oTilt.oMot_.oOut_.uiLastFaultState_ = oTilt.oMot_.oState_.uiDriveState_;
    state Fault_C
      entry:
      oTilt.oMot_.oState_.uiDriveState_ = 1003;
    (default) -> (junction 164)
    (junction 164) -> Fault_A [order 1] : [oTilt.oMot_.oState_.uiDriveState_>= 200]
    (junction 164) -> (junction 271) [order 2]
    (junction 271) -> Fault_C [order 2]
    (junction 271) -> Fault_B [order 1] : [oTilt.oMot_.oState_.uiDriveState_>= 1000]
    Fault_B -> Fault_C
  state Slave_start
    // Slave start is not applicable to position control.
    // Not a position control inverter; slave role is set: Perform a slave start (wait for the motor to 'somehow' reach a minimum speed, then jump on).
    entry:
    // We have to set one item aside; the desired rotation direction, as signalled by the sign of the current
    oTilt.oMot_.oState_.fForcedAngleStartDirection_ = single(oTilt.oMot_.oIn_.fIqSetpoint_ >= 0);
    // in other areas of MBD, we use oPitch.oMot_.oState_.oRampDataIqRef_.fRampOut_...should we here?
    // Don't actually turn on the output stage, but instead, monitor the motor feedback.
    // Once confident, perform a running start.
    // The rest is handled via state machine.
    oTilt.oMot_.oState_.uiDriveState_ = 220;
  state Enabled
    // [SZ]: Still need to model the setupForFlyingStart() function, which involves calling NEON sin/cos functions in Stateflow
    state Open_loop_start
      // Open loop start from standstill. Risky, and rough on hardware
      state Open_loop_start_A
        entry:
        oTilt.oMot_.oState_.oRampDataFluxFeedforwardGain_.fRampOut_ = 0.0;
        oTilt.oMot_.oState_.oRampDataOmegaERef_.fRampOut_ = 0.0;
        oTilt.oMot_.oState_.oRampDataIqRef_.fRampOut_ = 0.0;
        oTilt.oMot_.oState_.uiDriveState_ = 200;
      state Open_loop_start_B
        entry:
        oTilt.oMot_.oState_.uiDriveState_ = 205;
      (default) -> Open_loop_start_A
      Open_loop_start_A -> Open_loop_start_B [order 1] : [oTilt.oMot_.oParam_.uiAutomaticFanControlMode_ == 1]
    state Standing_start
      // ----- Set up for forced angle start ----
      state Store_reference
        // Store original references and ramp rates aside:
        entry:
        oTilt.oMot_.oState_.fForcedAngleStartOrigIRamp_ = oTilt.oMot_.oState_.oRampDataIqRef_.oParam_.fUpslope_;
        // TODO: whatabout downslope?
        oTilt.oMot_.oState_.fForcedAngleStartOrigOmega_ = oTilt.oMot_.oState_.oRampDataOmegaERef_.fSetpoint_;
        oTilt.oMot_.oState_.fForcedAngleStartOrigOmegaRamp_ = oTilt.oMot_.oState_.oRampDataOmegaERef_.oParam_.fUpslope_;
        // The downslope is never touched, as it doesn't matter for forced angle start
        oTilt.oMot_.oState_.uiForcedAngleStartOrigSpeedControllerActive_ = oTilt.oMot_.oState_.uiSpeedControllerActive_;
        // We have to set one item aside; the desired rotation direction, as signalled by the sign of the current
        oTilt.oMot_.oState_.fForcedAngleStartDirection_ = single(oTilt.oMot_.oState_.oRampDataIqRef_.fRampOut_ >= 0);
        // should this be oPitch.oMot_.oIn_.fIqSetpoint_ >= 0; ??
      state Global_signal
        // Signals to the rest of the program.
        oTilt.oMot_.oOut_.uiForcedAngle_ = 1;
        oTilt.oMot_.oState_.uiDriveState_ = 211;
      state Initialization
        // Set up initial values
        entry:
        // Delete this section once the uiForcedAngleStartParametersSet_ flag is working properly...
        oTilt.oMot_.oState_.fForcedAngleStartOrigIRamp_ = oTilt.oMot_.oState_.oRampDataIqRef_.oParam_.fUpslope_;
        // TODO: whatabout downslope?
        oTilt.oMot_.oState_.fForcedAngleStartOrigOmega_ = oTilt.oMot_.oState_.oRampDataOmegaERef_.fSetpoint_;
        oTilt.oMot_.oState_.fForcedAngleStartOrigOmegaRamp_ = oTilt.oMot_.oState_.oRampDataOmegaERef_.oParam_.fUpslope_;
        // The downslope is never touched, as it doesn't matter for forced angle start
        oTilt.oMot_.oState_.uiForcedAngleStartOrigSpeedControllerActive_ = oTilt.oMot_.oState_.uiSpeedControllerActive_;
        // We have to set one item aside; the desired rotation direction, as signalled by the sign of the current
        oTilt.oMot_.oState_.fForcedAngleStartDirection_ = single(oTilt.oMot_.oState_.oRampDataIqRef_.fRampOut_ >= 0);
        oTilt.oMot_.oState_.fIqRefBeforeRamp_ = oTilt.oMot_.oParam_.fForcedAngleIRef_;
        //oTilt.oMot_.oState_.oRampDataIqRef_.oParam_.fUpslope_ = oTilt.oMot_.oParam_.fForcedAngleIRamp_;
        oTilt.oMot_.oState_.oRampDataIqRef_.oParam_.fUpslope_ = oTilt.oMot_.oParam_.fForcedAngleIRamp_*10*(TARGET_CODE_GEN==0)+...
        oTilt.oMot_.oParam_.fForcedAngleIRamp_*(TARGET_CODE_GEN==1); // Adjust for 100 Hz state machine in simulation
        oTilt.oMot_.oState_.oRampDataIqRef_.oParam_.fDownslope_ = oTilt.oMot_.oState_.oRampDataIqRef_.oParam_.fUpslope_;
        //oTilt.oMot_.oState_.oRampDataOmegaERef_.oParam_.fUpslope_ = oTilt.oMot_.oParam_.fForcedAngleOmegaERamp_;
        oTilt.oMot_.oState_.oRampDataOmegaERef_.oParam_.fUpslope_ = oTilt.oMot_.oParam_.fForcedAngleOmegaERamp_*10*(TARGET_CODE_GEN==0)+...
        oTilt.oMot_.oParam_.fForcedAngleOmegaERamp_*(TARGET_CODE_GEN==1); // Adjust for 100 Hz state machine in simulation
        oTilt.oMot_.oState_.oRampDataOmegaERef_.fRampOut_ = 0.0F;
        oTilt.oMot_.oState_.oRampDataOmegaERef_.fSetpoint_ = 0.0F;
        oTilt.oMot_.oState_.oRampDataIqRef_.fRampOut_ = 0.0F;
        oTilt.oMot_.oState_.uiSpeedControllerActive_ = 0;
        oTilt.oMot_.oState_.uiForcedAngleStartParametersSet_ = 1;
        oTilt.oMot_.oState_.oRampDataFluxFeedforwardGain_.fRampOut_ = 0.0F;
      (default) -> Global_signal
      Global_signal -> (junction 233)
      (junction 233) -> Store_reference [order 1] : [!(oTilt.oMot_.oState_.uiForcedAngleStartParametersSet_ == 1)]
      (junction 233) -> Initialization [order 2]
      Store_reference -> Initialization
    state Half_duty_preset
      // Pre-set 50% duty
      entry:
      oTilt.oMot_.oOut_.uiPwmRequestFromMain_ = 1;
      oTilt.oMot_.oOut_.uiPwmDutyTicksFromMainA_ = uint32((oTilt.oMot_.oParam_.fPwmPeriodTicksMainloopFloat_)/2);
      oTilt.oMot_.oOut_.uiPwmDutyTicksFromMainB_ = uint32((oTilt.oMot_.oParam_.fPwmPeriodTicksMainloopFloat_)/2);
      oTilt.oMot_.oOut_.uiPwmDutyTicksFromMainC_ = uint32((oTilt.oMot_.oParam_.fPwmPeriodTicksMainloopFloat_)/2);
      oTilt.oIsr_.oParam_.oPiDataIq_.fState_ = 0.0F;
      oTilt.oIsr_.oParam_.oPiDataId_.fState_ = 0.0F;
      oTilt.oMot_.oParam_.oPiDataRpm_.fState_ = 0.0F;
      oTilt.oMot_.oParam_.oPid2DataRpmCtrl_.fState_ = 0.0F;
      oTilt.oMot_.oState_.oPosSensor_.oPidDataPosCtrl_.fState_ = 0.0F;
      oTilt.oMot_.oState_.oRampDataPos_.fRampOut_ = oTilt.oMot_.oState_.oPosSensor_.oGbx_.fCurrentOutputAngle_;
      // Prevent jerk motions on start up.
      // [SZ]: Moved here to avoid the "Unconditional Path Out of State with During Actions or Child States" warning
    state Release_gate_signal
      entry:
      oTilt.oIsr_.oState_.fOverspeedProtectionScaler_ = 1.0;
      oTilt.oMot_.oState_.oPosSensor_.iAngleElecFromSensorNumOfIdenticalValues_ = 0;
      // release gate signals
      oTilt.oMot_.oOut_.uiEnableGateDrive_ = 0x7;
      oTilt.oMot_.oOut_.uiCurrentControllerActive_ = 1; // Release control in main interrupt
    (default) -> (junction 184)
    (junction 184) -> Open_loop_start [order 2]
    (junction 184) -> Standing_start [order 1] : [oTilt.oMot_.oState_.uiForcedAngleStart_ == 1]
    Open_loop_start_A -> Half_duty_preset [order 2]
    Open_loop_start_B -> Half_duty_preset
    Initialization -> Half_duty_preset
    Half_duty_preset -> Release_gate_signal
  (default) -> Disabled
  Slave_start -> Disabled
  Position_hold_mode -> Disabled
  (junction 192) -> Disabled [order 1] : [oTilt.oMot_.oState_.uiDriveState_ < 101 || oTilt.oMot_.oState_.uiDriveState_ > 104]
  Disabled -> (junction 192) : [oTilt.oMot_.oOut_.uiEnable_ == 1]
  DC_undervoltage_trip -> Disabled : [oTilt.oIsr_.oState_.fUdcPostlpf_ > oTilt.oMot_.oParam_.fUdcMinTrip_]
  Enabled -> Disabled : [!(oTilt.oMot_.oOut_.uiEnable_ == 1)]
  (junction 192) -> Position_hold_mode [order 3] : [oTilt.oMot_.oParam_.iForcedPositionHoldMode_ == 1]
  (junction 192) -> DC_undervoltage_trip [order 2] : [oTilt.oIsr_.oState_.fUdcPostlpf_< oTilt.oMot_.oParam_.fUdcMinTrip_]
  (junction 192) -> Slave_start [order 4] : [oTilt.oMot_.oParam_.uiSlaveRole_ == 1 && !(oTilt.oMot_.oState_.oPosSensor_.iPosControlEnabled_ == 1)]
  (junction 192) -> (junction 273) [order 5]
  (junction 273) -> Enabled : [oTilt.oMot_.oState_.uiDriveState_ == 101 || oTilt.oMot_.oState_.uiDriveState_ == 103]
  data: TARGET_CODE_GEN parameter; oTilt data_store_memory
